simulink model "tunneldiode_sim"  (R2014a)
settings: Solver=ode45  StartTime=0.0  StopTime=15e-9  RelTol=1e-3
values from neighbouring files (symbols this model uses):
  C = 2    [E205_TeamProj.m]    (also in tunneldiode_GUI.m)
  L = 5    [E205_TeamProj.m]    (also in tunneldiode_GUI.m)
  R = 1.5    [E205_TeamProj.m]    (also in tunneldiode_GUI.m)
  tpulse = 40    [E205_TeamProj.m]    (also in tunneldiode_GUI.m = str2double(tpulse))
  Vmax = 1.65    [E205_TeamProj.m]    (also in tunneldiode_GUI.m = str2double(Vmax))
settings Model: Creator=Jessica  LastModifiedBy=Jessica

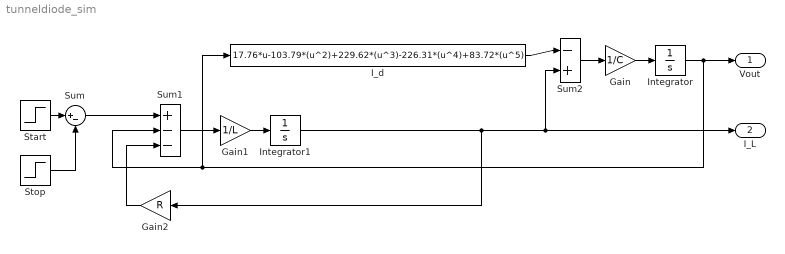
== system tunneldiode_sim ==
  Gain : Gain  Gain=1/C
  Gain1 : Gain  Gain=1/L
  Gain2 : Gain  Gain=R
  I_d : Fcn  Expr=17.76*u-103.79*(u^2)+229.62*(u^3)-226.31*(u^4)+83.72*(u^5)
  Integrator : Integrator
  Integrator1 : Integrator
  Start : Step  Time=0  After=Vmax  SampleTime=0
  Stop : Step  Time=tpulse  After=Vmax  SampleTime=0
  Sum : Sum  Inputs=|+-
  Sum1 : Sum  Inputs=|+|-|-
  Sum2 : Sum  Inputs=|-|+
  Vout : Outport
  I_L : Outport  Port=2
  wires:
  Gain/1 -> Integrator/1
  Sum2/1 -> Gain/1
  I_d/1 -> Sum2/1
  Integrator/1 -> Sum1/2, I_d/1, Vout/1
  Integrator1/1 -> Sum2/2, I_L/1, Gain2/1
  Gain1/1 -> Integrator1/1
  Sum1/1 -> Gain1/1
  Gain2/1 -> Sum1/3
  Start/1 -> Sum/1
  Sum/1 -> Sum1/1
  Stop/1 -> Sum/2
